simulink model "Simu_Cascade"  (R2022a)
settings: Solver=VariableStepAuto  StartTime=0.0  StopTime=100  RelTol=1e-3
libraries: slpidlib x1
settings Model: Creator=81909  LastModifiedBy=81909

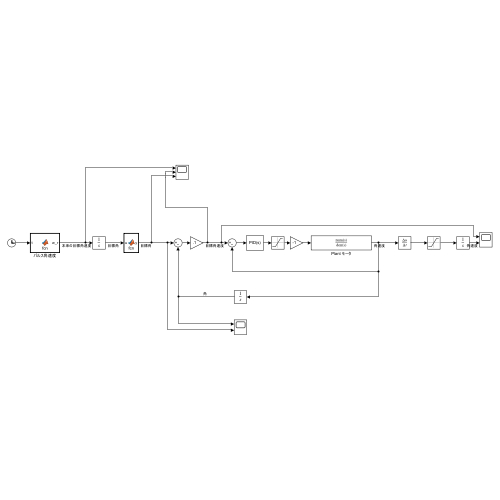
[thumbnail: Simulink's stored preview of the top-level diagram]
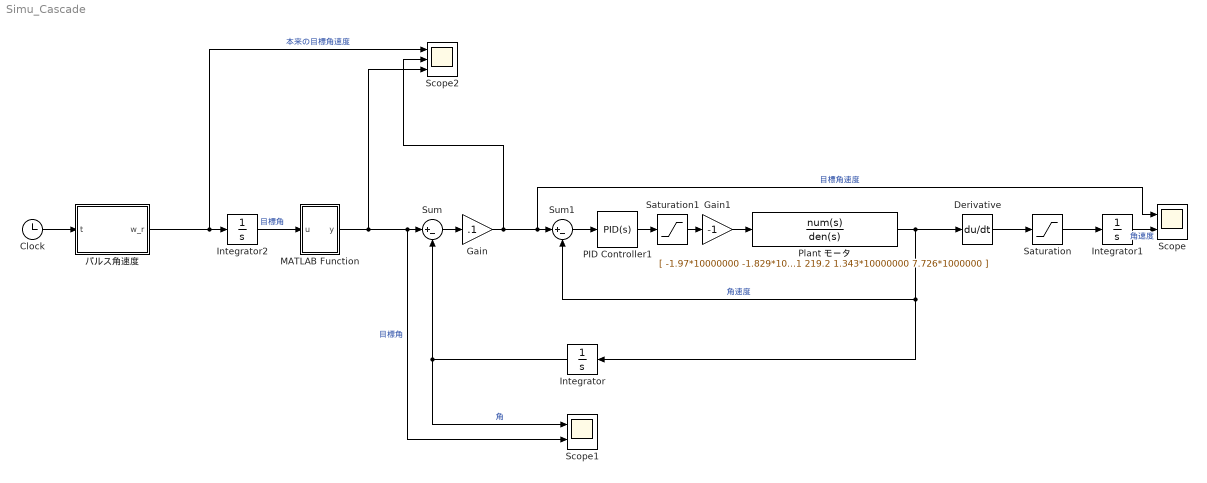
== system Simu_Cascade ==
  Clock : Clock
  Derivative : Derivative
  Gain : Gain  Gain=.1
  Gain1 : Gain  Gain=-1
  Integrator : Integrator
  Integrator1 : Integrator
  Integrator2 : Integrator
  MATLAB Function : MATLAB Function  TreatAsAtomicUnit=on
  PID Controller1 : slpidlib/PID Controller  Controller=PID  Form=Parallel  TimeDomain=Continuous-time  UseExternalTs=off  SampleTime=-1  IntegratorMethod=Forward Euler  FilterMethod=Forward Euler  ControllerParametersSource=internal  P=1  I=0  UseKiTs=off  D=0  N=100  UseFilter=on  TunerSelectOption=Transfer Function Based (PID Tuner App)  InitialConditionSource=internal  InitialConditionForIntegrator=0  InitialConditionForFilter=0  DifferentiatorICPrevScaledInput=0  ExternalReset=none  TrackingMode=off  Kt=1  LimitOutput=off  SatLimitsSource=internal  UpperSaturationLimit=inf  LowerSaturationLimit=-inf  LinearizeAsGain=on  AntiWindupMode=none  Kb=1  POutMin=[]  POutMax=[]  IOutMin=[]  IOutMax=[]  DOutMin=[]  DOutMax=[]  NOutMin=[]  NOutMax=[]  SumOutMin=[]  SumOutMax=[]  SaturationOutMin=[]  SaturationOutMax=[]  PParamMin=[]  PParamMax=[]  IParamMin=[]  IParamMax=[]  DParamMin=[]  DParamMax=[]  NParamMin=[]  NParamMax=[]  KbParamMin=[]  KbParamMax=[]  KtParamMin=[]  KtParamMax=[]  KbOutMin=[]  KbOutMax=[]  KtOutMin=[]  KtOutMax=[]  IntegratorOutMin=[]  IntegratorOutMax=[]  FilterOutMin=[]  FilterOutMax=[]  SumI1OutMin=[]  SumI1OutMax=[]  SumI2OutMin=[]  SumI2OutMax=[]  SumI3OutMin=[]  SumI3OutMax=[]  SumI4OutMin=[]  SumI4OutMax=[]  SumDOutMin=[]  SumDOutMax=[]  DifferentiatorOutMin=[]  DifferentiatorOutMax=[]  FilterDiffOutCoefMin=[]  FilterDiffOutCoefMax=[]  ReciprocalOutMin=[]  ReciprocalOutMax=[]  SumDenOutMin=[]  SumDenOutMax=[]  SumNumOutMin=[]  SumNumOutMax=[]  DivideOutMin=[]  DivideOutMax=[]  UdiffTsProdOutMin=[]  UdiffTsProdOutMax=[]  NTsProdOutMin=[]  NTsProdOutMax=[]  UintegralTsProdOutMin=[]  UintegralTsProdOutMax=[]  UngainTsProdOutMin=[]  UngainTsProdOutMax=[]  IntegratorContinuousStateAttributes=''  IntegratorStateMustResolveToSignalObject=off  IntegratorRTWStateStorageClass=Auto  FilterContinuousStateAttributes=''  FilterStateMustResolveToSignalObject=off  FilterRTWStateStorageClass=Auto  ParallelPVariant=InternalParameters  IdealPVariant=Disabled  IVariant=InternalParameters  DVariant=InternalParameters  IntegratorVariant=Continuous  SatVariant=Disabled  AWVariant=Passthrough  PCopyVariant=Disabled  TRVariant=Disabled  FdbkBlocksVariant=Forward  IdealPFdbkVariant=Disabled  SatFdbkVariant=Disabled  DerivativeFilterVariant=ContFilter  NVariant=InternalParameters  NCopyVariant=Disabled  FilterICVariant=InternalICsFilter  IntegratorICVariant=InternalICs  ExternalResetVariant=Disabled  TRSumVariant=Passthrough  SumFdbkVariant=Disabled  SumVariant=Sum_PID  TsampFilterVariant=InternalTs  TsampNgainVariant=Passthrough  TsampIntegralVariant=Passthrough  ExternalSaturationOutDataTypeStr=Inherit: Same as second input  aMode=0
  Plant モータ : TransferFcn  Numerator=[ -1.97*10000000 -1.829*10000000]  Denominator=[ 1 219.2 1.343*10000000 7.726*1000000 ]
  Saturation : Saturate  UpperLimit=43  LowerLimit=-44
  Saturation1 : Saturate  UpperLimit=12  LowerLimit=0
  Scope : Scope  NumInputPorts=2
  Scope1 : Scope  NumInputPorts=2
  Scope2 : Scope  NumInputPorts=3
  Sum : Sum  Inputs=|+-
  Sum1 : Sum  Inputs=|+-
  パルス角速度 : MATLAB Function  TreatAsAtomicUnit=on
  wires:
  Integrator2/1 -> MATLAB Function/1(u)  "目標角"
  Sum/1 -> Gain/1
  Sum1/1 -> PID Controller1/1
  Gain/1 -> Scope2/2, Scope/1, Sum1/1  "目標角速度"
  PID Controller1/1 -> Saturation1/1
  Plant モータ/1 -> Derivative/1, Sum1/2, Integrator/1  "角速度"
  Integrator/1 -> Scope1/1, Sum/2  "角"
  Derivative/1 -> Saturation/1
  Saturation/1 -> Integrator1/1
  Integrator1/1 -> Scope/2  "角速度"
  Saturation1/1 -> Gain1/1
  Gain1/1 -> Plant モータ/1
  パルス角速度/1(w_r) -> Scope2/1, Integrator2/1  "本来の目標角速度"
  Clock/1 -> パルス角速度/1(t)
  MATLAB Function/1(y) -> Scope2/3, Scope1/2, Sum/1  "目標角"

== matlab function Simu_Cascade/MATLAB Function ==
  data: u input; y output
function y = fcn(u)

y = (u - 360*floor(u/360));

== matlab function Simu_Cascade/パルス角速度 ==
  data: t input; w_r output
function w_r = fcn(t)
T = 0.4;

if(rem(t, T) <= 0.3)
    w_r = 15;
else
    w_r = 24;
end
